simulink model "ihc_nl_log"  (R2020b)
settings: Solver=FixedStepDiscrete  StartTime=0.0  StopTime=stopTime  FixedStep=2.0833333333333333e-05  RelTol=1e-3
values from neighbouring files (symbols this model uses):
  strength = (20.0e6)/(10^(corner/20))    (= 2000)    [modelparameters.m]
undefined symbols (not defined in the file or in its folder): mp
libraries: simulink x1
settings Model: Creator=Ross  LastModifiedBy=conno
settings DataIOCC: SaveOutput=off  SaveTime=off  ReturnWorkspaceOutputs=off
settings OptimizationCC: BlockReduction=off  ConditionallyExecuteInputs=off  DefaultParameterBehavior=Inlined
settings DebuggingCC: ReadBeforeWriteMsg=DisableAll  WriteAfterWriteMsg=DisableAll  WriteAfterReadMsg=DisableAll  AlgebraicLoopMsg=error  MultiTaskDSMMsg=none  SingleTaskRateTransMsg=error  PregeneratedLibrarySubsystemCodeDiagnostic=none  ArithmeticOperatorsInVariantConditions=warning
settings HardwareCC: ProdBitPerPointer=32  ProdBitPerSizeT=32  ProdBitPerPtrDiffT=32  ProdLargestAtomicFloat=None  ProdIntDivRoundTo=Undefined  ProdEndianess=Unspecified  ProdWordSize=32  ProdHWDeviceType=ASIC/FPGA->ASIC/FPGA  TargetBitPerPointer=64  TargetBitPerSizeT=64  TargetBitPerPtrDiffT=64  TargetLongLongMode=on  TargetIntDivRoundTo=Zero  TargetEndianess=LittleEndian  TargetWordSize=64  TargetHWDeviceType=Custom Processor->MATLAB Host Computer  ProdEqTarget=off
settings ModelReferenceCC: UpdateModelReferenceTargets=IfOutOfDate
settings SFSimCC: SFSimEcho=off  SimUseLocalCustomCode=off  CustomCodeUndefinedFunction=UseInterfaceOnly
settings RTWCC: RTWUseLocalCustomCode=off

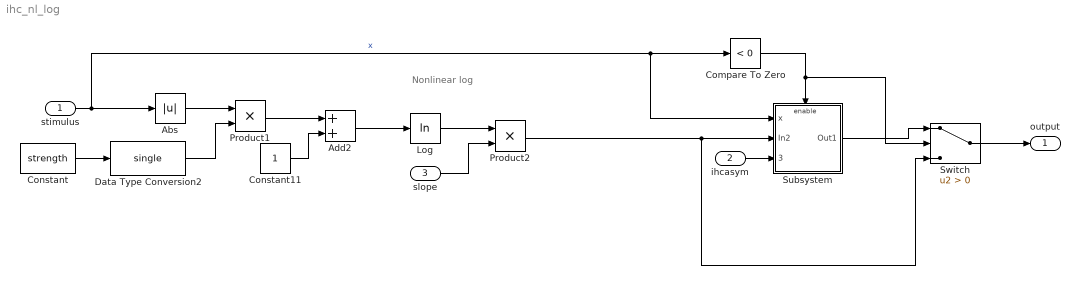
== system ihc_nl_log ==
  note: Nonlinear log
  stimulus : Inport  OutDataTypeStr=single  PortDimensions=1  SampleTime=[2.0833333333333333e-05,0]
  ihcasym : Inport  Port=2  OutDataTypeStr=single  PortDimensions=1  SampleTime=[2.0833333333333333e-05,0]
  slope : Inport  Port=3  OutDataTypeStr=single  PortDimensions=1  SampleTime=[2.0833333333333333e-05,0]
  Abs : Abs
  Add2 : Sum
  Compare To Zero : simulink/Logic and Bit Operations/Compare To Zero  relop=<  OutDataTypeStr=boolean
  Constant : Constant  Value=strength  SampleTime=mp.Ts_sim
  Constant11 : Constant  OutDataTypeStr=single  SampleTime=-1
  Data Type Conversion2 : DataTypeConversion  OutDataTypeStr=single
  Log : Math  Operator=log  SignedPower=on  SaturateOnIntegerOverflow=on
  Product1 : Product
  Product2 : Product
  Subsystem : Subsystem
  Switch : Switch  Criteria=u2 > Threshold
  output : Outport  OutDataTypeStr=single  PortDimensions=1  SampleTime=[2.0833333333333333e-05,0]  VectorParamsAs1DForOutWhenUnconnected=off
  wires:
  Switch/1 -> output/1
  Subsystem/1(Out1) -> Switch/1
  Compare To Zero/1 -> Subsystem/Enable, Switch/2
  Product2/1 -> Switch/3, Subsystem/2(In2)
  slope/1 -> Product2/2
  Log/1 -> Product2/1
  Add2/1 -> Log/1
  Product1/1 -> Add2/1
  Constant11/1 -> Add2/2
  Data Type Conversion2/1 -> Product1/2
  Abs/1 -> Product1/1
  stimulus/1 -> Subsystem/1(x), Compare To Zero/1, Abs/1  "x"
  ihcasym/1 -> Subsystem/3(ihcasym)
  Constant/1 -> Data Type Conversion2/1

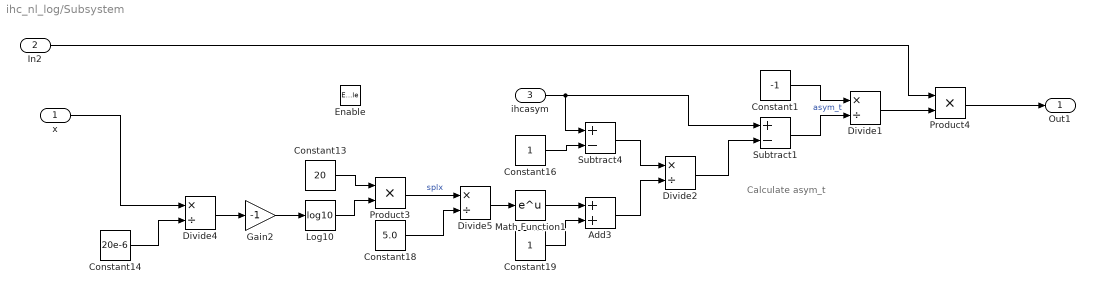
== system ihc_nl_log/Subsystem ==
  note: Calculate asym_t
  x : Inport
  In2 : Inport  Port=2
  ihcasym : Inport  Port=3
  Enable : EnablePort
  Add3 : Sum
  Constant1 : Constant  Value=-1  OutDataTypeStr=single  SampleTime=-1
  Constant13 : Constant  Value=20  OutDataTypeStr=single  SampleTime=-1
  Constant14 : Constant  Value=20e-6  OutDataTypeStr=single  SampleTime=-1
  Constant16 : Constant  OutDataTypeStr=single  SampleTime=-1
  Constant18 : Constant  Value=5.0  OutDataTypeStr=single  SampleTime=-1
  Constant19 : Constant  OutDataTypeStr=single  SampleTime=-1
  Divide{1..2,4..5} (4 alike) : Product  Inputs=*/  RndMeth=Zero  SaturateOnIntegerOverflow=on
  Gain2 : Gain  Gain=-1
  Log10 : Math  Operator=log10  SignedPower=on  SaturateOnIntegerOverflow=on
  Math Function1 : Math  SignedPower=on  SaturateOnIntegerOverflow=on
  Product3 : Product
  Product4 : Product
  Subtract1 : Sum  Inputs=+-
  Subtract4 : Sum  Inputs=+-
  Out1 : Outport  OutDataTypeStr=single  InitialOutput=[0]
  wires:
  Gain2/1 -> Log10/1
  Constant13/1 -> Product3/1
  Divide5/1 -> Math Function1/1
  Math Function1/1 -> Add3/1
  Product3/1 -> Divide5/1  "splx"
  Log10/1 -> Product3/2
  Constant14/1 -> Divide4/2
  Constant19/1 -> Add3/2
  Divide4/1 -> Gain2/1
  Constant18/1 -> Divide5/2
  Subtract4/1 -> Divide2/1
  ihcasym/1 -> Subtract1/1, Subtract4/1
  Add3/1 -> Divide2/2
  Divide2/1 -> Subtract1/2
  Subtract1/1 -> Divide1/2  "asym_t"
  Constant1/1 -> Divide1/1
  Constant16/1 -> Subtract4/2
  Divide1/1 -> Product4/2
  In2/1 -> Product4/1
  x/1 -> Divide4/1
  Product4/1 -> Out1/1
